simulink model "JABS_AutoSave_20200707_1052"  (R2018b)
settings: Solver=FixedStepDiscrete  StartTime=0.0  StopTime=10.0  FixedStep=0.01  RelTol=1e-3
(part 1 of 2)
settings Model: Creator=gaohang  LastModifiedBy=gaohang
settings OptimizationCC: BlockReduction=off  DefaultParameterBehavior=Inlined  UseDivisionForNetSlopeComputation=on  UseFloatMulNetSlope=on  DefaultUnderspecifiedDataType=single  UseSpecifiedMinMax=on  InlineInvariantSignals=on  PassReuseOutputArgsAs=Individual arguments  ZeroExternalMemoryAtStartup=off  ZeroInternalMemoryAtStartup=off  LifeSpan=inf  OptimizeBlockOrder=speed  DifferentSizesBufferReuse=on
settings DebuggingCC: SignalInfNanChecking=error  ReadBeforeWriteMsg=EnableAllAsError  WriteAfterWriteMsg=EnableAllAsError  WriteAfterReadMsg=EnableAllAsError  IntegerOverflowMsg=error  ParameterTunabilityLossMsg=error  UniqueDataStoreMsg=error  NonBusSignalsTreatedAsBus=error  IntegerSaturationMsg=error
settings ModelReferenceCC: UpdateModelReferenceTargets=IfOutOfDate
settings SFSimCC: SFSimEcho=off  CompileTimeRecursionLimit=0  MATLABDynamicMemAlloc=off
settings RTWCC: SystemTargetFile=autosar.tlc  GenCodeOnly=on  TemplateMakefile=ert_default_tmf  Description=AUTOSAR  GenerateReport=on  BuildConfiguration=Faster Runs  IncludeHyperlinkInReport=on  LaunchReport=on  GenerateTraceInfo=on  GenerateTraceReport=on  GenerateTraceReportSl=on  GenerateTraceReportSf=on  GenerateTraceReportEml=on  GenerateCodeMetricsReport=on
settings CodeAppCC: ForceParamTrailComments=on  IgnoreCustomStorageClasses=off  OperatorAnnotations=on  SimulinkDataObjDesc=on  SFDataObjDesc=on  MATLABFcnDesc=on  InsertBlockDesc=on  StateflowObjectComments=on  EnableCustomComments=on  ReqsInCode=on
settings STFCustomTargetCC: TargetLangStandard=C99 (ISO)  UtilityFuncGeneration=Shared location  MultiwordLength=256  ParMdlRefBuildCompliant=on  CompOptLevelCompliant=on  IncludeMdlTerminateFcn=off  CombineOutputUpdateFcns=on  CombineSignalStateStructs=on  SuppressErrorStatus=on  ERTCustomFileBanners=on  SupportNonFinite=off  SupportComplex=off  SupportContinuousTime=off  SupportNonInlinedSFcns=off  RemoveResetFunc=on  ParenthesesLevel=Maximum  CastingMode=Standards  MATLABClassNameForMDSCustomization=Simulink.SoftwareTarget.ERTCustomization  AutosarCompliant=on  UseToolchainInfoCompliant=on  GenerateSharedConstants=off  LookupTableObjectStructAxisOrder=2,1,3,4,...  LUTObjectStructOrderEvenSpacing=Size,Table,Breakpoints  SystemTargetFile=autosar.tlc
settings ERTTargetCC: TargetLangStandard=C99 (ISO)  UtilityFuncGeneration=Shared location  ConcurrentExecutionCompliant=off  IncludeMdlTerminateFcn=off  CombineSignalStateStructs=on  SuppressErrorStatus=on  SupportNonFinite=off  SupportComplex=off  ParenthesesLevel=Maximum  CastingMode=Standards  ModelStepFunctionPrototypeControlCompliant=off  CPPClassGenCompliant=off  AutosarCompliant=on  GenerateSharedConstants=off  LookupTableObjectStructAxisOrder=2,1,3,4,...  LUTObjectStructOrderEvenSpacing=Size,Table,Breakpoints  GenerateASAP2=on  InlinedParameterPlacement=NonHierarchical  ERTCustomFileTemplate=example_file_process.tlc  EnableSignedLeftShifts=off  EnableSignedRightShifts=off

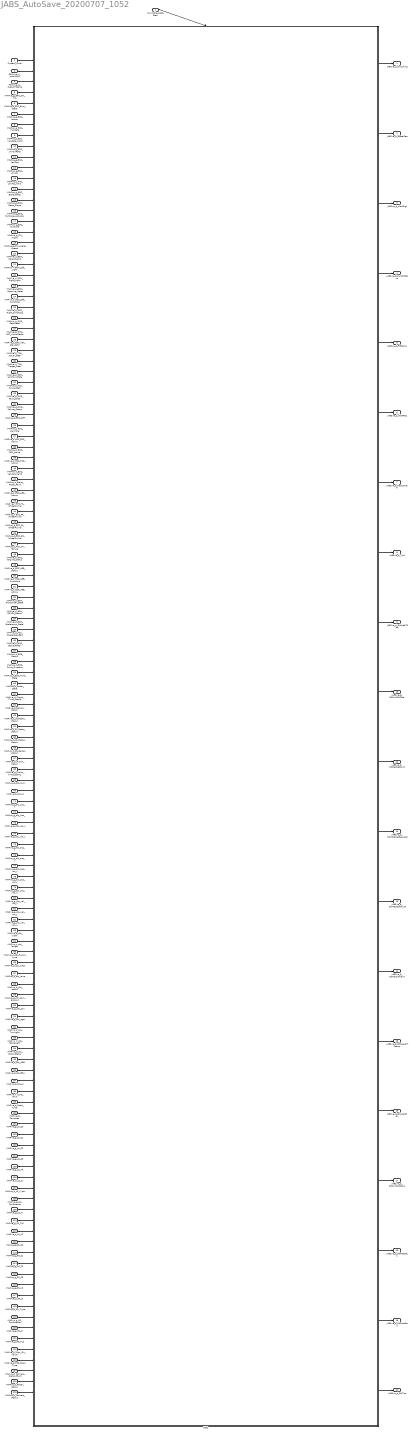
== system JABS_AutoSave_20200707_1052 ==
  Runnable_JABS_Step : Inport  SampleTime=0.01  OutputFunctionCall=on
  System_Clock : Inport  Port=2  OutDataTypeStr=UInt16
  FDMMve_d_JaFcnConf : Inport  Port=3  OutDataTypeStr=UInt16
  FDMMve_d_SignalTStamp : Inport  Port=4  OutDataTypeStr=UInt16
  IMAPve_g_EPS_SW_Trq : Inport  Port=5  OutDataTypeStr=T_M_Nm_Float32
  IMAPve_d_EPS_Error_State : Inport  Port=6  OutDataTypeStr=UInt16
  IMAPve_g_ESC_LatAcc : Inport  Port=7  OutDataTypeStr=T_M_Nm_Float32
  IMAPve_g_ESC_YawRate : Inport  Port=8  OutDataTypeStr=T_M_Nm_Float32
  IMAPve_d_ESC_YawRate_Valid : Inport  Port=9  OutDataTypeStr=UInt16
  IMAPve_g_ESC_UnYawRate : Inport  Port=10  OutDataTypeStr=T_M_Nm_Float32
  IMAPve_g_ESC_VehSpd : Inport  Port=11  OutDataTypeStr=T_M_Nm_Float32
  IMAPve_g_ESC_LonAcc : Inport  Port=12  OutDataTypeStr=T_M_Nm_Float32
  IMAPve_d_ESC_LonAcc_Valid : Inport  Port=13  OutDataTypeStr=UInt16
  IMAPve_g_ESC_Brake_Press : Inport  Port=14  OutDataTypeStr=T_M_Nm_Float32
  IMAPve_g_ESC_Static_Slope : Inport  Port=15  OutDataTypeStr=T_M_Nm_Float32
  IMAPve_g_ESC_DySlope_Accuracy : Inport  Port=16  OutDataTypeStr=T_M_Nm_Float32
  IMAPve_g_ESC_DySlope : Inport  Port=17  OutDataTypeStr=T_M_Nm_Float32
  IMAPve_g_SW_Angle : Inport  Port=18  OutDataTypeStr=T_M_Nm_Float32
  IMAPve_g_SW_Angle_Speed : Inport  Port=19  OutDataTypeStr=T_M_Nm_Float32
  IMAPve_d_BCM_HazardLamp : Inport  Port=20  OutDataTypeStr=UInt16
  IMAPve_d_BCM_Left_Light : Inport  Port=21  OutDataTypeStr=UInt16
  IMAPve_d_BCM_Right_Light : Inport  Port=22  OutDataTypeStr=UInt16
  IMAPve_d_BCM_Opening_State : Inport  Port=23  OutDataTypeStr=UInt16
  IMAPve_d_SCC_Left_SwitchSig : Inport  Port=24  OutDataTypeStr=UInt16
  IMAPve_d_SCC_Right_SwitchSig : Inport  Port=25  OutDataTypeStr=UInt16
  IMAPve_g_EMS_RealPedal : Inport  Port=26  OutDataTypeStr=T_M_Nm_Float32
  IMAPve_g_EMS_ACC_VirtualPedal : Inport  Port=27  OutDataTypeStr=T_M_Nm_Float32
  IMAPve_d_ESC_Veh_Standstill : Inport  Port=28  OutDataTypeStr=UInt16
  IMAPve_d_TCU_Actual_Gear : Inport  Port=29  OutDataTypeStr=UInt16
  IMAPve_d_TCU_Target_Gear : Inport  Port=30  OutDataTypeStr=UInt16
  IMAPve_d_BCM_Ignition_State : Inport  Port=31  OutDataTypeStr=UInt16
  IMAPve_d_ACU_Driver_Belt : Inport  Port=32  OutDataTypeStr=UInt16
  IMAPve_d_SWS_Fault_Code : Inport  Port=33  OutDataTypeStr=UInt16
  IMAPve_d_SWS_Failure_Status : Inport  Port=34  OutDataTypeStr=UInt16
  IMAPve_d_ESC_OFF : Inport  Port=35  OutDataTypeStr=UInt16
  IMAPve_d_ESC_AlarmSig : Inport  Port=36  OutDataTypeStr=UInt16
  IMAPve_d_ESC_ESC_Active : Inport  Port=37  OutDataTypeStr=UInt16
  IMAPve_d_ESC_MSR_Active : Inport  Port=38  OutDataTypeStr=UInt16
  IMAPve_d_ESC_TCS_Active : Inport  Port=39  OutDataTypeStr=UInt16
  IMAPve_d_ESC_VehSpd_Valid : Inport  Port=40  OutDataTypeStr=UInt16
  IMAPve_d_Brake_Pedal_Fault : Inport  Port=41  OutDataTypeStr=UInt16
  IMAPve_d_ESC_ABS_Active : Inport  Port=42  OutDataTypeStr=UInt16
  IMAPve_d_ESC_FL_WheelPulVal : Inport  Port=43  OutDataTypeStr=UInt16
  IMAPve_d_ESC_FR_WheelPulVal : Inport  Port=44  OutDataTypeStr=UInt16
  IMAPve_d_ESC_RL_WheelPulVal : Inport  Port=45  OutDataTypeStr=UInt16
  IMAPve_d_ESC_RR_WheelPulVal : Inport  Port=46  OutDataTypeStr=UInt16
  IMAPve_d_TCU_AT_Failure : Inport  Port=47  OutDataTypeStr=UInt16
  IMAPve_d_EMS_Engine_Status : Inport  Port=48  OutDataTypeStr=UInt16
  IMAPve_d_ESC_AEB_Status : Inport  Port=49  OutDataTypeStr=UInt16
  IMAPve_d_ESC_AEB_Available : Inport  Port=50  OutDataTypeStr=UInt16
  IMAPve_d_ESC_AEB_Active : Inport  Port=51  OutDataTypeStr=UInt16
  IMAPve_d_BCM_FrontWiper_State : Inport  Port=52  OutDataTypeStr=UInt16
  IMAPve_d_BCM_CHMSL_Status : Inport  Port=53  OutDataTypeStr=UInt16
  IMAPve_d_BCM_BrakeLamp_State : Inport  Port=54  OutDataTypeStr=UInt16
  IMAPve_d_ACU_Passenger_Belt : Inport  Port=55  OutDataTypeStr=UInt16
  IMAPve_d_EMS_Brake_Pedal : Inport  Port=56  OutDataTypeStr=UInt16
  IMAPve_d_EPB_Status : Inport  Port=57  OutDataTypeStr=UInt16
  IMAPve_d_ESC_Drive_Direction : Inport  Port=58  OutDataTypeStr=UInt16
  IMAPve_d_ESC_Hold_State : Inport  Port=59  OutDataTypeStr=UInt16
  IMAPve_d_Radar_State : Inport  Port=60  OutDataTypeStr=UInt16
  IMAPve_d_Signal_Time_Stamp : Inport  Port=61  OutDataTypeStr=UInt16
  IMAPve_d_Sensor_Status : Inport  Port=62  OutDataTypeStr=UInt16
  IMAPve_d_LF_Radar_Status : Inport  Port=63  OutDataTypeStr=UInt16
  IMAPve_d_RF_Radar_Status : Inport  Port=64  OutDataTypeStr=UInt16
  IMAPve_d_LR_Radar_Status : Inport  Port=65  OutDataTypeStr=UInt16
  IMAPve_d_RR_Radar_Status : Inport  Port=66  OutDataTypeStr=UInt16
  IMAPve_d_Fusion_Status : Inport  Port=67  OutDataTypeStr=UInt16
  IMAPve_g_Fusion_Time_Stamp : Inport  Port=68  OutDataTypeStr=T_M_Nm_Float32
  IMAPve_d_obj_Num : Inport  Port=69  OutDataTypeStr=UInt16
  IMAPva_d_obj_id : Inport  Port=70  OutDataTypeStr=UInt16  PortDimensions=40
  IMAPva_g_obj_pos_x : Inport  Port=71  OutDataTypeStr=T_M_Nm_Float32  PortDimensions=40
  IMAPva_g_obj_pos_y : Inport  Port=72  OutDataTypeStr=T_M_Nm_Float32  PortDimensions=40
  IMAPva_g_obj_vel_x : Inport  Port=73  OutDataTypeStr=T_M_Nm_Float32  PortDimensions=40
  IMAPva_g_obj_vel_y : Inport  Port=74  OutDataTypeStr=T_M_Nm_Float32  PortDimensions=40
  IMAPva_g_obj_acc_x : Inport  Port=75  OutDataTypeStr=T_M_Nm_Float32  PortDimensions=40
  IMAPva_g_obj_acc_y : Inport  Port=76  OutDataTypeStr=T_M_Nm_Float32  PortDimensions=40
  IMAPva_g_obj_pos_var_x : Inport  Port=77  OutDataTypeStr=T_M_Nm_Float32  PortDimensions=40
  IMAPva_g_obj_pos_var_y : Inport  Port=78  OutDataTypeStr=T_M_Nm_Float32  PortDimensions=40
  IMAPva_g_obj_pos_var_xy : Inport  Port=79  OutDataTypeStr=T_M_Nm_Float32  PortDimensions=40
  IMAPva_g_obj_vel_var_x : Inport  Port=80  OutDataTypeStr=T_M_Nm_Float32  PortDimensions=40
  IMAPva_g_obj_vel_var_y : Inport  Port=81  OutDataTypeStr=T_M_Nm_Float32  PortDimensions=40
  IMAPva_g_obj_vel_var_xy : Inport  Port=82  OutDataTypeStr=T_M_Nm_Float32  PortDimensions=40
  IMAPva_g_obj_width : Inport  Port=83  OutDataTypeStr=T_M_Nm_Float32  PortDimensions=40
  IMAPva_g_obj_length : Inport  Port=84  OutDataTypeStr=T_M_Nm_Float32  PortDimensions=40
  IMAPva_d_obj_fusion_type : Inport  Port=85  OutDataTypeStr=UInt16  PortDimensions=40
  IMAPva_d_obj_class : Inport  Port=86  OutDataTypeStr=UInt16  PortDimensions=40
  IMAPva_d_obj_lane : Inport  Port=87  OutDataTypeStr=UInt16  PortDimensions=40
  IMAPva_d_obj_status : Inport  Port=88  OutDataTypeStr=UInt16  PortDimensions=40
  IMAPva_d_obj_cam_asso_id : Inport  Port=89  OutDataTypeStr=UInt16  PortDimensions=40
  IMAPva_g_obj_con : Inport  Port=90  OutDataTypeStr=T_M_Nm_Float32  PortDimensions=40
  IMAPva_g_obj_age : Inport  Port=91  OutDataTypeStr=T_M_Nm_Float32  PortDimensions=40
  IMAPva_d_obj_TurnLight : Inport  Port=92  OutDataTypeStr=UInt16  PortDimensions=40
  IMAPva_d_obj_BrakeLight : Inport  Port=93  OutDataTypeStr=UInt16  PortDimensions=40
  IMAPva_d_obj_MotionStatus : Inport  Port=94  OutDataTypeStr=UInt16  PortDimensions=40
  IMAPva_d_obj_AEB : Inport  Port=95  OutDataTypeStr=UInt16  PortDimensions=40
  IMAPva_d_obj_ESA : Inport  Port=96  OutDataTypeStr=UInt16  PortDimensions=40
  IMAPva_d_obj_JA : Inport  Port=97  OutDataTypeStr=UInt16  PortDimensions=40
  IMAPve_d_Lane_Valid : Inport  Port=98  OutDataTypeStr=UInt16
  IMAPve_d_Road_Type : Inport  Port=99  OutDataTypeStr=UInt16
  IMAPve_d_ConsArea : Inport  Port=100  OutDataTypeStr=UInt16
  IMAPve_g_L0_C0 : Inport  Port=101  OutDataTypeStr=T_M_Nm_Float32
  IMAPve_g_L0_C1 : Inport  Port=102  OutDataTypeStr=T_M_Nm_Float32
  IMAPve_g_L0_C2 : Inport  Port=103  OutDataTypeStr=T_M_Nm_Float32
  IMAPve_g_L0_C3 : Inport  Port=104  OutDataTypeStr=T_M_Nm_Float32
  IMAPve_g_L0_VR : Inport  Port=105  OutDataTypeStr=T_M_Nm_Float32
  IMAPve_d_L0_Q : Inport  Port=106  OutDataTypeStr=UInt16
  IMAPve_d_L0_Type : Inport  Port=107  OutDataTypeStr=UInt16
  IMAPve_g_L0_Confidence : Inport  Port=108  OutDataTypeStr=T_M_Nm_Float32
  IMAPve_g_L0_W : Inport  Port=109  OutDataTypeStr=T_M_Nm_Float32
  IMAPve_g_L0_TLC : Inport  Port=110  OutDataTypeStr=T_M_Nm_Float32
  IMAPve_d_L0_LC : Inport  Port=111  OutDataTypeStr=UInt16
  IMAPve_g_R0_C0 : Inport  Port=112  OutDataTypeStr=T_M_Nm_Float32
  IMAPve_g_R0_C1 : Inport  Port=113  OutDataTypeStr=T_M_Nm_Float32
  IMAPve_g_R0_C2 : Inport  Port=114  OutDataTypeStr=T_M_Nm_Float32
  IMAPve_g_R0_C3 : Inport  Port=115  OutDataTypeStr=T_M_Nm_Float32
  IMAPve_g_R0_VR : Inport  Port=116  OutDataTypeStr=T_M_Nm_Float32
  IMAPve_d_R0_Q : Inport  Port=117  OutDataTypeStr=UInt16
  IMAPve_d_R0_Type : Inport  Port=118  OutDataTypeStr=UInt16
  IMAPve_g_R0_Confidence : Inport  Port=119  OutDataTypeStr=T_M_Nm_Float32
  IMAPve_g_R0_W : Inport  Port=120  OutDataTypeStr=T_M_Nm_Float32
  IMAPve_g_R0_TLC : Inport  Port=121  OutDataTypeStr=T_M_Nm_Float32
  IMAPve_d_Sign_ISA_Value : Inport  Port=122  OutDataTypeStr=UInt16
  IMAPve_d_TSR_Sign_Type : Inport  Port=123  OutDataTypeStr=UInt16
  IMAPve_d_Camera_Signal_Fault : Inport  Port=124  OutDataTypeStr=UInt16
  IMAPve_d_Radar_Status : Inport  Port=125  OutDataTypeStr=UInt16
  IMAPve_d_Camera_Status : Inport  Port=126  OutDataTypeStr=UInt16
  JABS : Subsystem  TreatAsAtomicUnit=on
  JABSve_d_Switching : Outport  OutDataTypeStr=UInt16
  JABSve_d_DecelReq : Outport  Port=2  OutDataTypeStr=T_M_Nm_Float32
  JABSve_d_AlertSign : Outport  Port=3  OutDataTypeStr=UInt16
  JABSve_d_SwitchStatus : Outport  Port=4  OutDataTypeStr=UInt16
  JABSve_d_FltStatus : Outport  Port=5  OutDataTypeStr=UInt16
  JABSve_d_AlertReq : Outport  Port=6  OutDataTypeStr=UInt16
  JABSve_d_HapticAlarm : Outport  Port=7  OutDataTypeStr=UInt16
  JABSve_d_Tips : Outport  Port=8  OutDataTypeStr=UInt16
  JABSve_d_DbPrefillReq : Outport  Port=9  OutDataTypeStr=UInt16
  JABSve_d_DbFunFARCSta : Outport  Port=10  OutDataTypeStr=UInt16
  JABSve_d_DbDecSetpoint : Outport  Port=11  OutDataTypeStr=T_M_Nm_Float32
  JABSve_d_DbMDDdecRequest : Outport  Port=12  OutDataTypeStr=UInt16
  JABSve_d_DbMDDdecType : Outport  Port=13  OutDataTypeStr=UInt16
  JABSve_d_DbHapticAlarm : Outport  Port=14  OutDataTypeStr=UInt16
  JABSve_d_DbSignalTStamp : Outport  Port=15  OutDataTypeStr=UInt16
  JABSve_d_DbAlertSign : Outport  Port=16  OutDataTypeStr=UInt16
  JABSve_d_DbSwitchStatus : Outport  Port=17  OutDataTypeStr=UInt16
  JABSve_d_DbFltStatus : Outport  Port=18  OutDataTypeStr=UInt16
  JABSve_d_DbAlertReq : Outport  Port=19  OutDataTypeStr=UInt16
  JABSve_d_DbTips : Outport  Port=20  OutDataTypeStr=UInt16
  wires:
  System_Clock/1 -> JABS/1(System_Clock)
  FDMMve_d_JaFcnConf/1 -> JABS/2(FDMMve_d_JaFcnConf)
  FDMMve_d_SignalTStamp/1 -> JABS/3(FDMMve_d_SignalTStamp)
  IMAPve_g_EPS_SW_Trq/1 -> JABS/4(IMAPve_g_EPS_SW_Trq)
  IMAPve_d_EPS_Error_State/1 -> JABS/5(IMAPve_d_EPS_Error_State)
  IMAPve_g_ESC_LatAcc/1 -> JABS/6(IMAPve_g_ESC_LatAcc)
  IMAPve_g_ESC_YawRate/1 -> JABS/7(IMAPve_g_ESC_YawRate)
  IMAPve_d_ESC_YawRate_Valid/1 -> JABS/8(IMAPve_d_ESC_YawRate_Valid)
  IMAPve_g_ESC_UnYawRate/1 -> JABS/9(IMAPve_g_ESC_UnYawRate)
  IMAPve_g_ESC_VehSpd/1 -> JABS/10(IMAPve_g_ESC_VehSpd)
  IMAPve_g_ESC_LonAcc/1 -> JABS/11(IMAPve_g_ESC_LonAcc)
  IMAPve_d_ESC_LonAcc_Valid/1 -> JABS/12(IMAPve_d_ESC_LonAcc_Valid)
  IMAPve_g_ESC_Brake_Press/1 -> JABS/13(IMAPve_g_ESC_Brake_Press)
  IMAPve_g_ESC_Static_Slope/1 -> JABS/14(IMAPve_g_ESC_Static_Slope)
  IMAPve_g_ESC_DySlope_Accuracy/1 -> JABS/15(IMAPve_g_ESC_DySlope_Accuracy)
  IMAPve_g_ESC_DySlope/1 -> JABS/16(IMAPve_g_ESC_DySlope)
  IMAPve_g_SW_Angle/1 -> JABS/17(IMAPve_g_SW_Angle)
  IMAPve_g_SW_Angle_Speed/1 -> JABS/18(IMAPve_g_SW_Angle_Speed)
  IMAPve_d_BCM_HazardLamp/1 -> JABS/19(IMAPve_d_BCM_HazardLamp)
  IMAPve_d_BCM_Left_Light/1 -> JABS/20(IMAPve_d_BCM_Left_Light)
  IMAPve_d_BCM_Right_Light/1 -> JABS/21(IMAPve_d_BCM_Right_Light)
  IMAPve_d_BCM_Opening_State/1 -> JABS/22(IMAPve_d_BCM_Opening_State)
  IMAPve_d_SCC_Left_SwitchSig/1 -> JABS/23(IMAPve_d_SCC_Left_SwitchSig)
  IMAPve_d_SCC_Right_SwitchSig/1 -> JABS/24(IMAPve_d_SCC_Right_SwitchSig)
  IMAPve_g_EMS_RealPedal/1 -> JABS/25(IMAPve_g_EMS_RealPedal)
  IMAPve_g_EMS_ACC_VirtualPedal/1 -> JABS/26(IMAPve_g_EMS_ACC_VirtualPedal)
  IMAPve_d_ESC_Veh_Standstill/1 -> JABS/27(IMAPve_d_ESC_Veh_Standstill)
  IMAPve_d_TCU_Actual_Gear/1 -> JABS/28(IMAPve_d_TCU_Actual_Gear)
  IMAPve_d_TCU_Target_Gear/1 -> JABS/29(IMAPve_d_TCU_Target_Gear)
  IMAPve_d_BCM_Ignition_State/1 -> JABS/30(IMAPve_d_BCM_Ignition_State)
  IMAPve_d_ACU_Driver_Belt/1 -> JABS/31(IMAPve_d_ACU_Driver_Belt)
  IMAPve_d_SWS_Fault_Code/1 -> JABS/32(IMAPve_d_SWS_Fault_Code)
  IMAPve_d_SWS_Failure_Status/1 -> JABS/33(IMAPve_d_SWS_Failure_Status)
  IMAPve_d_ESC_OFF/1 -> JABS/34(IMAPve_d_ESC_OFF)
  IMAPve_d_ESC_AlarmSig/1 -> JABS/35(IMAPve_d_ESC_AlarmSig)
  IMAPve_d_ESC_ESC_Active/1 -> JABS/36(IMAPve_d_ESC_ESC_Active)
  IMAPve_d_ESC_MSR_Active/1 -> JABS/37(IMAPve_d_ESC_MSR_Active)
  IMAPve_d_ESC_TCS_Active/1 -> JABS/38(IMAPve_d_ESC_TCS_Active)
  IMAPve_d_ESC_VehSpd_Valid/1 -> JABS/39(IMAPve_d_ESC_VehSpd_Valid)
  IMAPve_d_Brake_Pedal_Fault/1 -> JABS/40(IMAPve_d_Brake_Pedal_Fault)
  IMAPve_d_ESC_ABS_Active/1 -> JABS/41(IMAPve_d_ESC_ABS_Active)
  IMAPve_d_ESC_FL_WheelPulVal/1 -> JABS/42(IMAPve_d_ESC_FL_WheelPulVal)
  IMAPve_d_ESC_FR_WheelPulVal/1 -> JABS/43(IMAPve_d_ESC_FR_WheelPulVal)
  IMAPve_d_ESC_RL_WheelPulVal/1 -> JABS/44(IMAPve_d_ESC_RL_WheelPulVal)
  IMAPve_d_ESC_RR_WheelPulVal/1 -> JABS/45(IMAPve_d_ESC_RR_WheelPulVal)
  IMAPve_d_TCU_AT_Failure/1 -> JABS/46(IMAPve_d_TCU_AT_Failure)
  IMAPve_d_EMS_Engine_Status/1 -> JABS/47(IMAPve_d_EMS_Engine_Status)
  IMAPve_d_ESC_AEB_Status/1 -> JABS/48(IMAPve_d_ESC_AEB_Status)
  IMAPve_d_ESC_AEB_Available/1 -> JABS/49(IMAPve_d_ESC_AEB_Available)
  IMAPve_d_ESC_AEB_Active/1 -> JABS/50(IMAPve_d_ESC_AEB_Active)
  IMAPve_d_BCM_FrontWiper_State/1 -> JABS/51(IMAPve_d_BCM_FrontWiper_State)
  IMAPve_d_BCM_CHMSL_Status/1 -> JABS/52(IMAPve_d_BCM_CHMSL_Status)
  IMAPve_d_BCM_BrakeLamp_State/1 -> JABS/53(IMAPve_d_BCM_BrakeLamp_State)
  IMAPve_d_ACU_Passenger_Belt/1 -> JABS/54(IMAPve_d_ACU_Passenger_Belt)
  IMAPve_d_EMS_Brake_Pedal/1 -> JABS/55(IMAPve_d_EMS_Brake_Pedal)
  IMAPve_d_EPB_Status/1 -> JABS/56(IMAPve_d_EPB_Status)
  IMAPve_d_ESC_Drive_Direction/1 -> JABS/57(IMAPve_d_ESC_Drive_Direction)
  IMAPve_d_ESC_Hold_State/1 -> JABS/58(IMAPve_d_ESC_Hold_State)
  IMAPve_d_Radar_State/1 -> JABS/59(IMAPve_d_Radar_State)
  IMAPve_d_Signal_Time_Stamp/1 -> JABS/60(IMAPve_d_Signal_Time_Stamp)
  IMAPve_d_Sensor_Status/1 -> JABS/61(IMAPve_d_Sensor_Status)
  IMAPve_d_LF_Radar_Status/1 -> JABS/62(IMAPve_d_LF_Radar_Status)
  IMAPve_d_RF_Radar_Status/1 -> JABS/63(IMAPve_d_RF_Radar_Status)
  IMAPve_d_LR_Radar_Status/1 -> JABS/64(IMAPve_d_LR_Radar_Status)
  IMAPve_d_RR_Radar_Status/1 -> JABS/65(IMAPve_d_RR_Radar_Status)
  IMAPve_d_Fusion_Status/1 -> JABS/66(IMAPve_d_Fusion_Status)
  IMAPve_g_Fusion_Time_Stamp/1 -> JABS/67(IMAPve_g_Fusion_Time_Stamp)
  IMAPve_d_obj_Num/1 -> JABS/68(IMAPve_d_obj_Num)
  IMAPva_d_obj_id/1 -> JABS/69(IMAPva_d_obj_id)
  IMAPva_g_obj_pos_x/1 -> JABS/70(IMAPva_g_obj_pos_x)
  IMAPva_g_obj_pos_y/1 -> JABS/71(IMAPva_g_obj_pos_y)
  IMAPva_g_obj_vel_x/1 -> JABS/72(IMAPva_g_obj_vel_x)
  IMAPva_g_obj_vel_y/1 -> JABS/73(IMAPva_g_obj_vel_y)
  IMAPva_g_obj_acc_x/1 -> JABS/74(IMAPva_g_obj_acc_x)
  IMAPva_g_obj_acc_y/1 -> JABS/75(IMAPva_g_obj_acc_y)
  IMAPva_g_obj_pos_var_x/1 -> JABS/76(IMAPva_g_obj_pos_var_x)
  IMAPva_g_obj_pos_var_y/1 -> JABS/77(IMAPva_g_obj_pos_var_y)
  IMAPva_g_obj_pos_var_xy/1 -> JABS/78(IMAPva_g_obj_pos_var_xy)
  IMAPva_g_obj_vel_var_x/1 -> JABS/79(IMAPva_g_obj_vel_var_x)
  IMAPva_g_obj_vel_var_y/1 -> JABS/80(IMAPva_g_obj_vel_var_y)
  IMAPva_g_obj_vel_var_xy/1 -> JABS/81(IMAPva_g_obj_vel_var_xy)
  IMAPva_g_obj_width/1 -> JABS/82(IMAPva_g_obj_width)
  IMAPva_g_obj_length/1 -> JABS/83(IMAPva_g_obj_length)
  IMAPva_d_obj_fusion_type/1 -> JABS/84(IMAPva_d_obj_fusion_type)
  IMAPva_d_obj_class/1 -> JABS/85(IMAPva_d_obj_class)
  IMAPva_d_obj_lane/1 -> JABS/86(IMAPva_d_obj_lane)
  IMAPva_d_obj_status/1 -> JABS/87(IMAPva_d_obj_status)
  IMAPva_d_obj_cam_asso_id/1 -> JABS/88(IMAPva_d_obj_cam_asso_id)
  IMAPva_g_obj_con/1 -> JABS/89(IMAPva_g_obj_con)
  IMAPva_g_obj_age/1 -> JABS/90(IMAPva_g_obj_age)
  IMAPva_d_obj_TurnLight/1 -> JABS/91(IMAPva_d_obj_TurnLight)
  IMAPva_d_obj_BrakeLight/1 -> JABS/92(IMAPva_d_obj_BrakeLight)
  IMAPva_d_obj_MotionStatus/1 -> JABS/93(IMAPva_d_obj_MotionStatus)
  IMAPva_d_obj_AEB/1 -> JABS/94(IMAPva_d_obj_AEB)
  IMAPva_d_obj_ESA/1 -> JABS/95(IMAPva_d_obj_ESA)
  IMAPva_d_obj_JA/1 -> JABS/96(IMAPva_d_obj_JA)
  IMAPve_d_Lane_Valid/1 -> JABS/97(IMAPve_d_Lane_Valid)
  IMAPve_d_Road_Type/1 -> JABS/98(IMAPve_d_Road_Type)
  IMAPve_d_ConsArea/1 -> JABS/99(IMAPve_d_ConsArea)
  IMAPve_g_L0_C0/1 -> JABS/100(IMAPve_g_L0_C0)
  IMAPve_g_L0_C1/1 -> JABS/101(IMAPve_g_L0_C1)
  IMAPve_g_L0_C2/1 -> JABS/102(IMAPve_g_L0_C2)
  IMAPve_g_L0_C3/1 -> JABS/103(IMAPve_g_L0_C3)
  IMAPve_g_L0_VR/1 -> JABS/104(IMAPve_g_L0_VR)
  IMAPve_d_L0_Q/1 -> JABS/105(IMAPve_d_L0_Q)
  IMAPve_d_L0_Type/1 -> JABS/106(IMAPve_d_L0_Type)
  IMAPve_g_L0_Confidence/1 -> JABS/107(IMAPve_g_L0_Confidence)
  IMAPve_g_L0_W/1 -> JABS/108(IMAPve_g_L0_W)
  IMAPve_g_L0_TLC/1 -> JABS/109(IMAPve_g_L0_TLC)
  IMAPve_d_L0_LC/1 -> JABS/110(IMAPve_d_L0_LC)
  IMAPve_g_R0_C0/1 -> JABS/111(IMAPve_g_R0_C0)
  IMAPve_g_R0_C1/1 -> JABS/112(IMAPve_g_R0_C1)
  IMAPve_g_R0_C2/1 -> JABS/113(IMAPve_g_R0_C2)
  IMAPve_g_R0_C3/1 -> JABS/114(IMAPve_g_R0_C3)
  IMAPve_g_R0_VR/1 -> JABS/115(IMAPve_g_R0_VR)
  IMAPve_d_R0_Q/1 -> JABS/116(IMAPve_d_R0_Q)
  IMAPve_d_R0_Type/1 -> JABS/117(IMAPve_d_R0_Type)
  IMAPve_g_R0_Confidence/1 -> JABS/118(IMAPve_g_R0_Confidence)
  IMAPve_g_R0_W/1 -> JABS/119(IMAPve_g_R0_W)
  IMAPve_g_R0_TLC/1 -> JABS/120(IMAPve_g_R0_TLC)
  IMAPve_d_Sign_ISA_Value/1 -> JABS/121(IMAPve_d_Sign_ISA_Value)
  IMAPve_d_TSR_Sign_Type/1 -> JABS/122(IMAPve_d_TSR_Sign_Type)
  IMAPve_d_Camera_Signal_Fault/1 -> JABS/123(IMAPve_d_Camera_Signal_Fault)
  IMAPve_d_Radar_Status/1 -> JABS/124(IMAPve_d_Radar_Status)
  IMAPve_d_Camera_Status/1 -> JABS/125(IMAPve_d_Camera_Status)
  Runnable_JABS_Step/1 -> JABS/Trigger
  JABS/1(JABSve_d_Switching) -> JABSve_d_Switching/1
  JABS/2(JABSve_d_DecelReq) -> JABSve_d_DecelReq/1
  JABS/3(JABSve_d_AlertSign) -> JABSve_d_AlertSign/1
  JABS/4(JABSve_d_SwitchStatus) -> JABSve_d_SwitchStatus/1
  JABS/5(JABSve_d_FltStatus) -> JABSve_d_FltStatus/1
  JABS/6(JABSve_d_AlertReq) -> JABSve_d_AlertReq/1
  JABS/7(JABSve_d_HapticAlarm) -> JABSve_d_HapticAlarm/1
  JABS/8(JABSve_d_Tips) -> JABSve_d_Tips/1
  JABS/9(JABSve_d_DbPrefillReq) -> JABSve_d_DbPrefillReq/1
  JABS/10(JABSve_d_DbFunFARCSta) -> JABSve_d_DbFunFARCSta/1
  JABS/11(JABSve_d_DbDecSetpoint) -> JABSve_d_DbDecSetpoint/1
  JABS/12(JABSve_d_DbMDDdecRequest) -> JABSve_d_DbMDDdecRequest/1
  JABS/13(JABSve_d_DbMDDdecType) -> JABSve_d_DbMDDdecType/1
  JABS/14(JABSve_d_DbHapticAlarm) -> JABSve_d_DbHapticAlarm/1
  JABS/15(JABSve_d_DbSignalTStamp) -> JABSve_d_DbSignalTStamp/1
  JABS/16(JABSve_d_DbAlertSign) -> JABSve_d_DbAlertSign/1
  JABS/17(JABSve_d_DbSwitchStatus) -> JABSve_d_DbSwitchStatus/1
  JABS/18(JABSve_d_DbFltStatus) -> JABSve_d_DbFltStatus/1
  JABS/19(JABSve_d_DbAlertReq) -> JABSve_d_DbAlertReq/1
  JABS/20(JABSve_d_DbTips) -> JABSve_d_DbTips/1
